simulink model "pt8612pll_3"  (Simulink 5.0)
settings: Solver=ode45  StartTime=0.0  StopTime=100  RelTol=1e-8  AbsTol=1e-11
values from neighbouring files (symbols this model uses):
  C = 680e-9    (= 6.8e-07)    [PT8612PLLinit.m]    (also in PT8612PLLinit_2.m; PT8612PLLinit_3.m; PT8612PLLinit_4.m; colorimetry_rom.m = [[CrCgCb(1) 0 0];[0 CrCgCb(2) 0];[0 0 CrCgCb(3)]])
  fvcxo = 148.5e6/1.001    (= 148351648.352)    [PT8612PLLinit.m]    (also in PT8612PLLinit_2.m; PT8612PLLinit_3.m; PT8612PLLinit_4.m)
  Gdd = 1/8    (= 0.125)    [PT8612PLLinit_2.m]    (also in PT8612PLLinit_3.m = 0)
  Gid = Gi*Tlfi    (= 2.15703703704e-05)    [PT8612PLLinit_2.m]    (also in PT8612PLLinit_3.m = 1.68518518519e-05)
  Gpd = 0.25    [PT8612PLLinit_2.m]    (also in PT8612PLLinit_3.m = 0.0002)
  Kvcxo = 90e-6    (= 9e-05)    [PT8612PLLinit.m]    (also in PT8612PLLinit_2.m; PT8612PLLinit_3.m; PT8612PLLinit_4.m)
  Mdac = 1    [PT8612PLLinit_3.m]    (also in PT8612PLLinit_4.m)
  Nbit = 12    [PT8612PLLinit_2.m]    (also in PT8612PLLinit_3.m)
  Nfodiv = 500*4    (= 2000)    [PT8612PLLinit_2.m]    (also in PT8612PLLinit_3.m; PT8612PLLinit_4.m = 500000)
  R = 100e3    (= 100000)    [PT8612PLLinit.m]    (also in PT8612PLLinit_2.m = 220000; PT8612PLLinit_3.m = 82000; PT8612PLLinit_4.m = 200000; combi_signal.m = [R;ones(red_heigth,spl)])
  Tlfd = 1000*500/fvcxo    (= 0.00337037037037)    [PT8612PLLinit_2.m]    (also in PT8612PLLinit_3.m = 0.000337037037037)
  Tlfi = 128*500/fvcxo    (= 0.000431407407407)    [PT8612PLLinit_2.m]    (also in PT8612PLLinit_3.m = 0.0337037037037)
  Tsphase = 1/fvcxo*Nfodiv    (= 1.34814814815e-05)    [PT8612PLLinit_2.m]    (also in PT8612PLLinit_3.m)
  Vcc = 3.3    [PT8612PLLinit_2.m]    (also in PT8612PLLinit_3.m; PT8612PLLinit_4.m)
libraries: simulink x3
settings Model: LastModifiedBy=thh

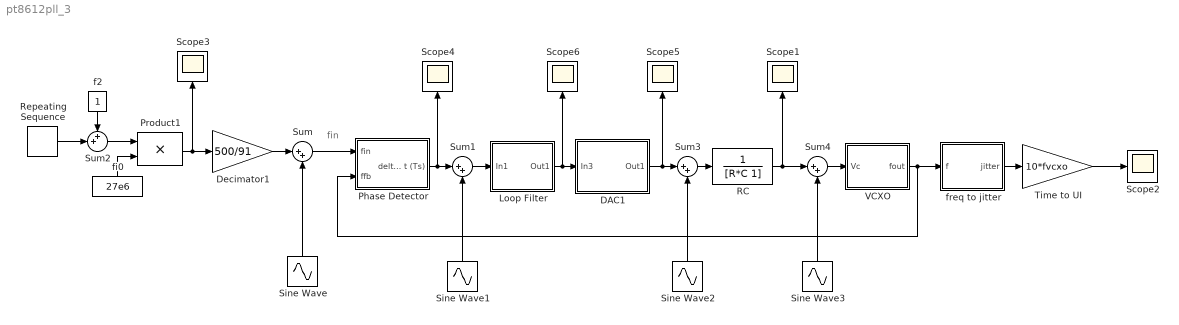
== system pt8612pll_3 ==
  note: fin
  DAC1 : Subsystem
  Decimator1 : Gain  Gain=500/91  SaturateOnIntegerOverflow=on
  Loop Filter : Subsystem
  Phase Detector : Subsystem
  Product1 : Product  SaturateOnIntegerOverflow=on
  RC : TransferFcn  Denominator=[R*C 1]
  Repeating Sequence : simulink/Sources/Repeating Sequence  rep_seq_t=[0 4 4 1000]  rep_seq_y=[1 1 0 0]*20e-6
  Scope{1..6} (6 alike) : Scope
      Scope1 settings: Orientation=up  TimeRange=10  YMin=1.24775  YMax=1.2525
      Scope2 settings: TimeRange=10  YMin=-1500  YMax=1500  SaveName=ScopeData3
      Scope3 settings: Orientation=up  YMin=2.565e+007  YMax=2.835e+007  SaveName=ScopeData4
      Scope4 settings: Orientation=up  TimeRange=10  YMin=0  YMax=350
      Scope5 settings: Orientation=up  TimeRange=10  YMin=-0.175  YMax=0.175  SaveName=ScopeData5
      Scope6 settings: Orientation=up  TimeRange=10  YMax=25  SaveName=ScopeData6
  Sine Wave : Sin  Orientation=up  Amplitude=0%1e-6  Frequency=100  SampleTime=0
  Sine Wave1 : Sin  Orientation=up  Amplitude=0  Frequency=1000  SampleTime=0
  Sine Wave2 : Sin  Orientation=up  Amplitude=0  SampleTime=0
  Sine Wave3 : Sin  Orientation=up  Amplitude=0  Frequency=100  SampleTime=0
  Sum{,1,3..4} (4 alike) : Sum  Inputs=|++  SaturateOnIntegerOverflow=on
  Sum2 : Sum  Inputs=++|  SaturateOnIntegerOverflow=on
  Time to UI : Gain  Gain=10*fvcxo  SaturateOnIntegerOverflow=on
  VCXO : Subsystem
  f2 : Constant  Orientation=down
  fi0 : Constant  Orientation=up  Value=27e6
  freq to jitter : Subsystem
  wires:
  Phase Detector/1(delta t (Ts)) -> Scope4/1, Sum1/1
  VCXO/1(fout) -> freq to jitter/1(f), Phase Detector/2(ffb)
  Product1/1 -> Scope3/1, Decimator1/1
  f2/1 -> Sum2/1
  Sum2/1 -> Product1/1
  Repeating Sequence/1 -> Sum2/2
  Loop Filter/1(Out1) -> DAC1/1(In3), Scope6/1
  freq to jitter/1(jitter) -> Time to UI/1
  fi0/1 -> Product1/2
  Time to UI/1 -> Scope2/1
  Sum/1 -> Phase Detector/1(fin)
  Decimator1/1 -> Sum/1
  Sine Wave/1 -> Sum/2
  DAC1/1(Out1) -> Scope5/1, Sum3/1
  RC/1 -> Scope1/1, Sum4/1
  Sum1/1 -> Loop Filter/1(In1)
  Sine Wave1/1 -> Sum1/2
  Sum3/1 -> RC/1
  Sine Wave2/1 -> Sum3/2
  Sum4/1 -> VCXO/1(Vc)
  Sine Wave3/1 -> Sum4/2

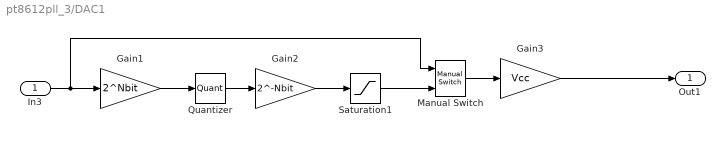
== system pt8612pll_3/DAC1 ==
  In3 : Inport
  Gain1 : Gain  Gain=2^Nbit  SaturateOnIntegerOverflow=on
  Gain2 : Gain  Gain=2^-Nbit  SaturateOnIntegerOverflow=on
  Gain3 : Gain  Gain=Vcc  SaturateOnIntegerOverflow=on
  Manual Switch : simulink/Signal Routing/Manual Switch  sw=1  action=0
  Quantizer : Quantizer  QuantizationInterval=1
  Saturation1 : Saturate  UpperLimit=Mdac  LowerLimit=0
  Out1 : Outport
  wires:
  In3/1 -> Gain1/1, Manual Switch/1
  Quantizer/1 -> Gain2/1
  Gain1/1 -> Quantizer/1
  Gain2/1 -> Saturation1/1
  Manual Switch/1 -> Gain3/1
  Gain3/1 -> Out1/1
  Saturation1/1 -> Manual Switch/2

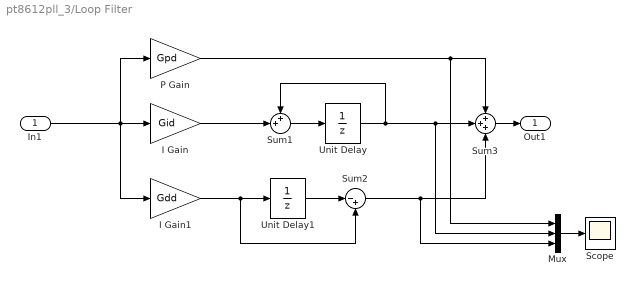
== system pt8612pll_3/Loop Filter ==
  In1 : Inport
  I Gain : Gain  Gain=Gid  SaturateOnIntegerOverflow=on
  I Gain1 : Gain  Gain=Gdd  SaturateOnIntegerOverflow=on
  Mux : Mux  Inputs=3
  P Gain : Gain  Gain=Gpd  SaturateOnIntegerOverflow=on
  Scope : Scope
      settings: YMin=0  YMax=0.07  SaveName=ScopeData2
  Sum1 : Sum  Inputs=++|  SaturateOnIntegerOverflow=on
  Sum2 : Sum  Inputs=|-+  SaturateOnIntegerOverflow=on
  Sum3 : Sum  Inputs=+++  SaturateOnIntegerOverflow=on
  Unit Delay : UnitDelay  SampleTime=Tlfi
  Unit Delay1 : UnitDelay  SampleTime=Tlfd
  Out1 : Outport
  wires:
  P Gain/1 -> Sum3/1, Mux/1
  Sum3/1 -> Out1/1
  Mux/1 -> Scope/1
  I Gain1/1 -> Unit Delay1/1, Sum2/2
  Unit Delay/1 -> Sum3/2, Mux/2, Sum1/1
  Sum1/1 -> Unit Delay/1
  I Gain/1 -> Sum1/2
  Unit Delay1/1 -> Sum2/1
  Sum2/1 -> Sum3/3, Mux/3
  In1/1 -> I Gain/1, P Gain/1, I Gain1/1

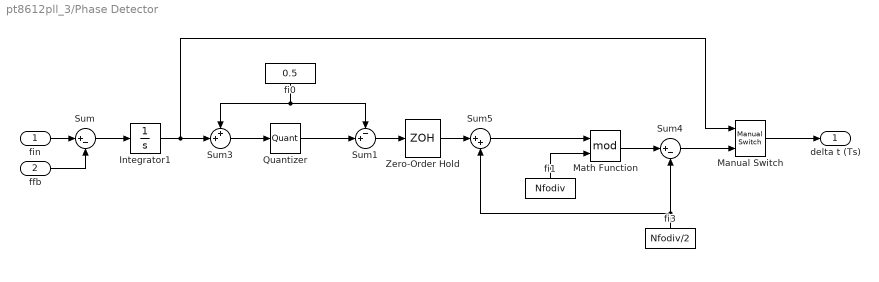
== system pt8612pll_3/Phase Detector ==
  fin : Inport
  ffb : Inport  Port=2
  Integrator1 : Integrator
  Manual Switch : simulink/Signal Routing/Manual Switch  sw=0  action=0
  Math Function : Math  Operator=mod
  Quantizer : Quantizer  QuantizationInterval=1
  Sum : Sum  Inputs=|+-  SaturateOnIntegerOverflow=on
  Sum1 : Sum  Inputs=-+|  SaturateOnIntegerOverflow=on
  Sum3 : Sum  Inputs=++|  SaturateOnIntegerOverflow=on
  Sum4 : Sum  Inputs=|+-  SaturateOnIntegerOverflow=on
  Sum5 : Sum  Inputs=|++  SaturateOnIntegerOverflow=on
  Zero-Order Hold : ZeroOrderHold  SampleTime=Tsphase
  fi0 : Constant  Orientation=down  Value=0.5
  fi1 : Constant  Orientation=up  Value=Nfodiv
  fi3 : Constant  Orientation=up  Value=Nfodiv/2
  delta t (Ts) : Outport
  wires:
  Sum/1 -> Integrator1/1
  fin/1 -> Sum/1
  ffb/1 -> Sum/2
  Sum3/1 -> Quantizer/1
  Integrator1/1 -> Sum3/2, Manual Switch/1
  Quantizer/1 -> Sum1/2
  fi0/1 -> Sum3/1, Sum1/1
  fi1/1 -> Math Function/2
  Sum1/1 -> Zero-Order Hold/1
  Zero-Order Hold/1 -> Sum5/1
  Sum5/1 -> Math Function/1
  fi3/1 -> Sum4/2, Sum5/2
  Math Function/1 -> Sum4/1
  Manual Switch/1 -> delta t (Ts)/1
  Sum4/1 -> Manual Switch/2

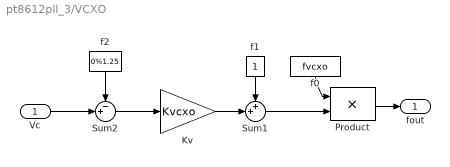
== system pt8612pll_3/VCXO ==
  Vc : Inport
  Kv : Gain  Gain=Kvcxo  SaturateOnIntegerOverflow=on
  Product : Product  SaturateOnIntegerOverflow=on
  Sum1 : Sum  Inputs=++|  SaturateOnIntegerOverflow=on
  Sum2 : Sum  Inputs=-+|  SaturateOnIntegerOverflow=on
  f0 : Constant  Orientation=down  Value=fvcxo
  f1 : Constant  Orientation=down
  f2 : Constant  Orientation=down  Value=0%1.25
  fout : Outport
  wires:
  f0/1 -> Product/1
  f1/1 -> Sum1/1
  Sum1/1 -> Product/2
  Kv/1 -> Sum1/2
  Product/1 -> fout/1
  Sum2/1 -> Kv/1
  Vc/1 -> Sum2/2
  f2/1 -> Sum2/1

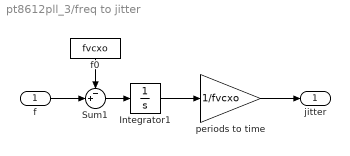
== system pt8612pll_3/freq to jitter ==
  f : Inport
  Integrator1 : Integrator
  Sum1 : Sum  Inputs=-+|  SaturateOnIntegerOverflow=on
  f0 : Constant  Orientation=down  Value=fvcxo
  periods to time : Gain  Gain=1/fvcxo  SaturateOnIntegerOverflow=on
  jitter : Outport
  wires:
  Integrator1/1 -> periods to time/1
  Sum1/1 -> Integrator1/1
  f0/1 -> Sum1/1
  f/1 -> Sum1/2
  periods to time/1 -> jitter/1
